simulink model "SmartCar2"  (R2022a)
settings: Solver=FixedStepDiscrete  StartTime=0.0  StopTime=10.0  FixedStep=0.1  RelTol=1e-3  EnableMultiTasking=on
settings Model: Creator=ASUS  LastModifiedBy=ASUS
settings SolverCC: AlgebraicLoopSolver=TrustRegion  AutoInsertRateTranBlk=on
settings DataIOCC: LimitDataPoints=on
settings OptimizationCC: DefaultParameterBehavior=Inlined  EnhancedBackFolding=on  PassReuseOutputArgsAs=Individual arguments  ZeroExternalMemoryAtStartup=off  ZeroInternalMemoryAtStartup=off  OptimizeBlockOrder=speed  DifferentSizesBufferReuse=on  OptimizationCustomize=off  EfficientTunableParamExpr=on
settings DebuggingCC: ParameterTunabilityLossMsg=error  UnconnectedInputMsg=warning  UnconnectedOutputMsg=warning  UnconnectedLineMsg=warning  AllowSymbolicDim=off  SFUnexpectedBacktrackingDiag=warning  SFNoUnconditionalDefaultTransitionDiag=warning  SFExecutionAtInitializationDiag=none  ArithmeticOperatorsInVariantConditions=warning
settings SFSimCC: SimUseLocalCustomCode=off  MATLABDynamicMemAlloc=off  CustomCodeUndefinedFunction=UseInterfaceOnly
settings RTWCC: SystemTargetFile=ert.tlc  TemplateMakefile=ert_default_tmf  RTWUseLocalCustomCode=off  DLArmComputeVersion=19.05
settings CodeAppCC: ForceParamTrailComments=on  IgnoreCustomStorageClasses=off  OperatorAnnotations=on  SimulinkDataObjDesc=on  SFDataObjDesc=on  InsertBlockDesc=on
settings ERTTargetCC: GenerateSampleERTMain=on  InlinedParameterPlacement=NonHierarchical  ERTCustomFileTemplate=example_file_process.tlc
settings ConfigComp: CovMetricSettings=dw  CovSaveCumulativeToWorkspaceVar=on  CovSaveSingleToWorkspaceVar=on  CovExternalEMLEnable=off  CovSFcnEnable=off

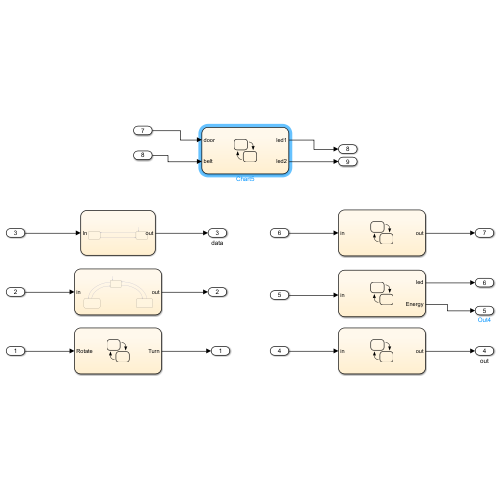
[thumbnail: Simulink's stored preview of the top-level diagram]
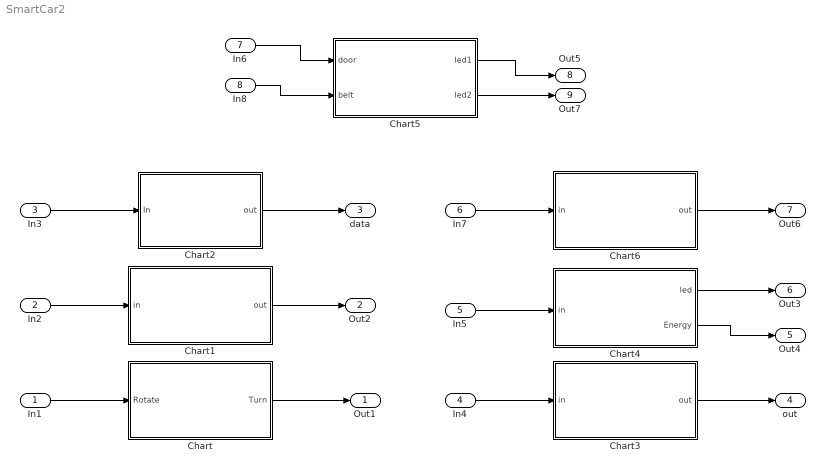
== system SmartCar2 ==
  In1 : Inport
  In2 : Inport  Port=2
  In3 : Inport  Port=3
  In4 : Inport  Port=4
  In5 : Inport  Port=5
  In7 : Inport  Port=6
  In6 : Inport  Port=7
  In8 : Inport  Port=8
  Chart : Stateflow chart  TreatAsAtomicUnit=on
  Chart1 : Stateflow chart  TreatAsAtomicUnit=on
  Chart2 : Stateflow chart  TreatAsAtomicUnit=on
  Chart3 : Stateflow chart  TreatAsAtomicUnit=on
  Chart4 : Stateflow chart  TreatAsAtomicUnit=on
  Chart5 : Stateflow chart  TreatAsAtomicUnit=on
  Chart6 : Stateflow chart  TreatAsAtomicUnit=on
  Out1 : Outport
  Out2 : Outport  Port=2
  data : Outport  Port=3
  out : Outport  Port=4
  Out4 : Outport  Port=5
  Out3 : Outport  Port=6
  Out6 : Outport  Port=7
  Out5 : Outport  Port=8
  Out7 : Outport  Port=9
  wires:
  In1/1 -> Chart/1(Rotate)
  Chart/1(Turn) -> Out1/1
  In2/1 -> Chart1/1(in)
  Chart1/1(out) -> Out2/1
  In3/1 -> Chart2/1(In)
  Chart2/1(out) -> data/1
  In4/1 -> Chart3/1(in)
  In5/1 -> Chart4/1(in)
  Chart4/2(Energy) -> Out4/1
  Chart3/1(out) -> out/1
  Chart4/1(led) -> Out3/1
  Chart6/1(out) -> Out6/1
  In7/1 -> Chart6/1(in)
  Chart5/2(led2) -> Out7/1
  Chart5/1(led1) -> Out5/1
  In8/1 -> Chart5/2(belt)
  In6/1 -> Chart5/1(door)

== stateflow chart SmartCar2/Chart4 ==
  state S1
  state S2
  state S3
  state S4
  (default) -> S1
  S1 -> S2 : [in<5]{Energy = 75 , led = 1}
  S2 -> S3 : [in<2.5]{Energy = 25 , led = 2}
  S3 -> S4 : [in==0]{Energy = 0 , led = 3}
  data: led output; Energy output; in input

== stateflow chart SmartCar2/Chart5 ==
  state S2
  state S1
  state S4
  state S3
  (default) -> S1
  S2 -> S1 [order 2] : [door == 1]{led1 = 1}
  S4 -> S2 [order 2] : [belt == 0]{led2 = 0}
  S2 -> S4 [order 1] : [belt == 0]{led2 = 0}
  S3 -> S1 [order 1] : [belt == 0]{led2 = 0}
  S1 -> S3 : [belt == 1]{led2 = 1}
  S3 -> S4 [order 2] : [door == 0]{led1 = 0}
  S4 -> S3 [order 1] : [door == 1]{led1 = 1}
  data: led1 output; door input; belt input; led2 output

== stateflow chart SmartCar2/Chart6 ==
  state S1
  state S2
  (default) -> S1
  S1 -> S2 : [in == 0]{out = 1}
  S2 -> S1 : [in > 0]{out = 0}
  data: out output; in input

== stateflow chart SmartCar2/Chart1 ==
  state S1
  state S3
  state S2
  (default) -> S1
  S2 -> S1 : [in == 0]{out = 0}
  S1 -> S3 [order 1] : [in < 0]{out = -1}
  S1 -> S2 [order 2] : [in > 0]{out = 1}
  S3 -> S1 : [in == 0]{out = 0}
  data: in input; out output

== stateflow chart SmartCar2/Chart2 ==
  state S2
  state S1
  (default) -> S1
  S1 -> S2 : [In == 1]{out = 1}
  S2 -> S1 : [In == 0]{out = 0}
  data: In input; out output

== stateflow chart SmartCar2/Chart ==
  state S2
  state S1
  state S4
  state S3
  (default) -> S1
  S2 -> S1 [order 2] : [Rotate == 0]{Turn = 0}
  S1 -> S2 [order 2] : [Rotate == 1]{Turn = 90}
  S4 -> S2 [order 2] : [Rotate == 0]{Turn = 90}
  S2 -> S4 [order 1] : [Rotate == 1]{Turn = 180}
  S3 -> S1 [order 1] : [Rotate == 1]{Turn = 0}
  S1 -> S3 [order 1] : [Rotate == 0]{Turn = -90}
  S3 -> S4 [order 2] : [Rotate == 0]{Turn = 180}
  S4 -> S3 [order 1] : [Rotate == 1]{Turn = -90}
  data: Turn output; Rotate input

== stateflow chart SmartCar2/Chart3 ==
  state S1
  state S2
  state S3
  state S4
  state S5
  S1 -> S2 [order 2] : [in < 50]{out = 0.25}
  (default) -> S1
  S2 -> S3 : [in<20]{out = 0.5}
  S3 -> S4 [order 2] : [in < 10]{out = 0.75}
  S4 -> S5 [order 2] : [in < 5]{out = 1}
  S4 -> S1 [order 1] : [in > 50]{out = 0}
  S3 -> S1 [order 1] : [in > 50]{out = 0}
  S1 -> S2 [order 1] : [in > 50]{out = 0}
  S5 -> S1 : [in > 50]{out = 0}
  data: in input; out output
